simulink model "IKS02A1_VL53L1A1_Both_ROS_fromworkspace_2025b_forstudents"  (R2025b)
settings: Solver=FixedStepAuto  StartTime=0.0  StopTime=sensorLog.GT_time.time(end)  FixedStep=1/200  RelTol=1e-3
settings Model: Creator=abich  LastModifiedBy=ashra

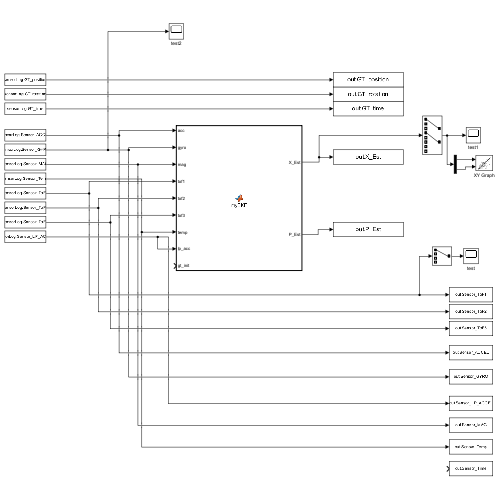
[thumbnail: Simulink's stored preview of the top-level diagram]
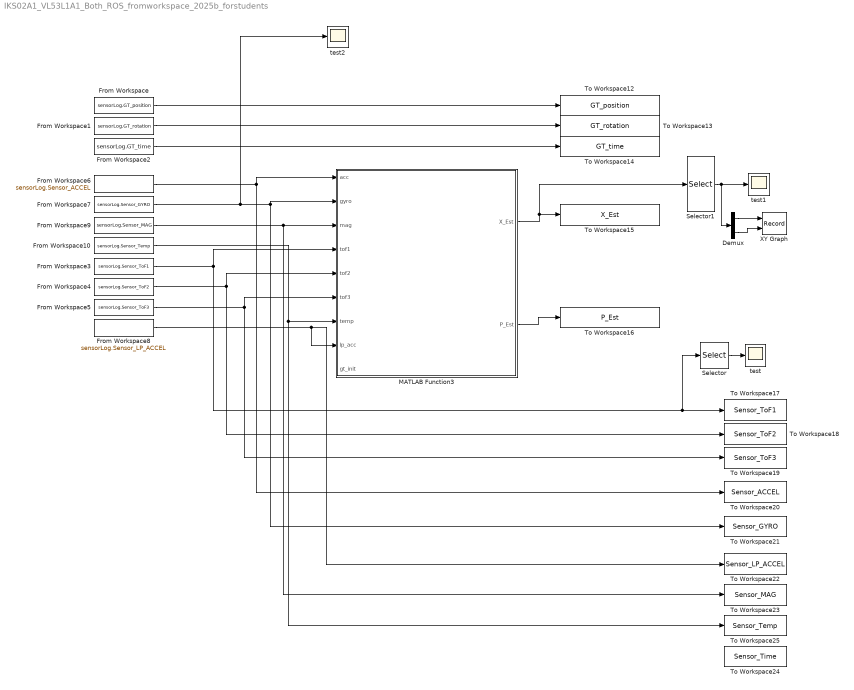
== system IKS02A1_VL53L1A1_Both_ROS_fromworkspace_2025b_forstudents ==
  Demux : Demux  Outputs=2
  From Workspace : FromWorkspace  VariableName=sensorLog.GT_position  SampleTime=1/200  OutputAfterFinalValue=Holding final value
  From Workspace1 : FromWorkspace  VariableName=sensorLog.GT_rotation  SampleTime=1/200  OutputAfterFinalValue=Holding final value
  From Workspace10 : FromWorkspace  VariableName=sensorLog.Sensor_Temp  SampleTime=1/200  OutputAfterFinalValue=Holding final value
  From Workspace2 : FromWorkspace  VariableName=sensorLog.GT_time  SampleTime=1/200  OutputAfterFinalValue=Holding final value
  From Workspace3 : FromWorkspace  VariableName=sensorLog.Sensor_ToF1  SampleTime=1/200  OutputAfterFinalValue=Holding final value
  From Workspace4 : FromWorkspace  VariableName=sensorLog.Sensor_ToF2  SampleTime=1/200  OutputAfterFinalValue=Holding final value
  From Workspace5 : FromWorkspace  VariableName=sensorLog.Sensor_ToF3  SampleTime=1/200  OutputAfterFinalValue=Holding final value
  From Workspace6 : FromWorkspace  VariableName=sensorLog.Sensor_ACCEL  SampleTime=1/200  OutputAfterFinalValue=Holding final value
  From Workspace7 : FromWorkspace  VariableName=sensorLog.Sensor_GYRO  SampleTime=1/200  OutputAfterFinalValue=Holding final value
  From Workspace8 : FromWorkspace  VariableName=sensorLog.Sensor_LP_ACCEL  SampleTime=1/200  OutputAfterFinalValue=Holding final value
  From Workspace9 : FromWorkspace  VariableName=sensorLog.Sensor_MAG  SampleTime=1/200  OutputAfterFinalValue=Holding final value
  MATLAB Function3 : MATLAB Function  TreatAsAtomicUnit=on
  Selector : Selector  InputPortWidth=4  IndexOptions=Index vector (dialog)  Indices=[1]  OutputSizes=1
  Selector1 : Selector  InputPortWidth=8  IndexOptions=Index vector (dialog)  Indices=[1 4]  OutputSizes=1
  To Workspace12 : ToWorkspace  VariableName=GT_position  SaveFormat=Structure With Time  SampleTime=1/200
  To Workspace13 : ToWorkspace  VariableName=GT_rotation  SaveFormat=Structure With Time  SampleTime=1/200
  To Workspace14 : ToWorkspace  VariableName=GT_time  SaveFormat=Structure With Time  SampleTime=1/200
  To Workspace15 : ToWorkspace  VariableName=X_Est  SaveFormat=Structure With Time  SampleTime=1/200
  To Workspace16 : ToWorkspace  VariableName=P_Est  SaveFormat=Structure With Time  SampleTime=1/200
  To Workspace17 : ToWorkspace  VariableName=Sensor_ToF1  SaveFormat=Structure With Time  SampleTime=1/200
  To Workspace18 : ToWorkspace  VariableName=Sensor_ToF2  SaveFormat=Structure With Time  SampleTime=1/200
  To Workspace19 : ToWorkspace  VariableName=Sensor_ToF3  SaveFormat=Structure With Time  SampleTime=1/200
  To Workspace20 : ToWorkspace  VariableName=Sensor_ACCEL  SaveFormat=Structure With Time  SampleTime=1/200
  To Workspace21 : ToWorkspace  VariableName=Sensor_GYRO  SaveFormat=Structure With Time  SampleTime=1/200
  To Workspace22 : ToWorkspace  VariableName=Sensor_LP_ACCEL  SaveFormat=Structure With Time  SampleTime=1/200
  To Workspace23 : ToWorkspace  VariableName=Sensor_MAG  SaveFormat=Structure With Time  SampleTime=1/200
  To Workspace24 : ToWorkspace  VariableName=Sensor_Time  SaveFormat=Structure With Time  SampleTime=1/200
  To Workspace25 : ToWorkspace  VariableName=Sensor_Temp  SaveFormat=Structure With Time  SampleTime=1/200
  XY Graph : Record  NumPorts=2.0  FileSettingsInternal="{\"entries\":[{\"content\":{\"excelSettings\":{\"content\":{},\"type\":\"Streamout.ExcelSettings\"},\"parquetSettings\":{\"content\":{},\"type\":\"Streamout.ParquetSettings\"}},\"type\":\"Streamout.FileSettingStorage\",\"uuid\":\"\"}],\"packageUris\":[\"http:\\/\\/schema.mathworks.com\\/mf0\\/streamout_blocks\\/R2020a\"],\"version\":\"1.0\"}"  FrameSettings=[0, 0]  Layout=[1 1]  SignalsInternal="{\"entries\":[{\"content\":{\"signals\":[{\"content\":{\"blockPath\":[],\"dimensions\":[1],\"domain\":\"\",\"lineColor\":\"#a2142f\",\"plots\":[ 1 ],\"port\":1,\"sid\":[\"\"],\"signalID\":1,\"signalName\":\"Demux:1\"},\"type\":\"RecordBlkView.Signal\",\"uuid\":\"\"},{\"content\":{\"blockPath\":[],\"dimensions\":[1],\"domain\":\"\",\"lineColor\":\"#139fff\",\"plots\":[ 1 ],\"port\":2,\"sid\":[\"\"],\"signalID\":2,\"signalName\":\"Demux:2\"},\"type\":\"RecordBlkView.Signal\",\"uuid\":\"\"}]},\"type\":\"RecordBlkView.InputSignals\",\"uuid\":\"\"}],\"packageUris\":[\"http:\\/\\/schema.mathworks.com\\/mf0\\/streamout_blocks\\/R2020a\"],\"version\":\"1.0\"}"  VisualizationBindings="{\"xyplotplugin\":{\"info\":[{\"series\":[{\"bindingParametersList\":[{\"parameter\":\"X-Axis\",\"signalID\":1,\"signalName\":\"Demux:1\"},{\"parameter\":\"Y-Axis\",\"signalID\":2,\"signalName\":\"Demux:2\"}],\"seriesID\":0}],\"subplotID\":1}]}}"  CompatibilityTag=XY
  test : Scope
      settings: ActiveDisplayYMinimum=-1  ActiveDisplayYMaximum=1
  test1 : Scope
      settings: ActiveDisplayYMinimum=-1.7865963660348574  ActiveDisplayYMaximum=1.7799074794929401
  test2 : Scope
      settings: ActiveDisplayYMinimum=-0.15108420974985681  ActiveDisplayYMaximum=0.16772460685752888  DataLoggingVariableName=ScopeData2
  wires:
  From Workspace4/1 -> To Workspace18/1, MATLAB Function3/5(tof2)
  From Workspace6/1 -> To Workspace20/1, MATLAB Function3/1(acc)
  From Workspace9/1 -> To Workspace23/1, MATLAB Function3/3(mag)
  From Workspace10/1 -> To Workspace25/1, MATLAB Function3/7(temp)
  From Workspace2/1 -> To Workspace14/1
  From Workspace5/1 -> To Workspace19/1, MATLAB Function3/6(tof3)
  From Workspace/1 -> To Workspace12/1
  MATLAB Function3/1(X_Est) -> Selector1/1, To Workspace15/1
  From Workspace8/1 -> To Workspace22/1, MATLAB Function3/8(lp_acc)
  From Workspace3/1 -> Selector/1, To Workspace17/1, MATLAB Function3/4(tof1)
  From Workspace1/1 -> To Workspace13/1
  From Workspace7/1 -> test2/1, To Workspace21/1, MATLAB Function3/2(gyro)
  MATLAB Function3/2(P_Est) -> To Workspace16/1
  Selector/1 -> test/1
  Selector1/1 -> Demux/1, test1/1
  Demux/1 -> XY Graph/1
  Demux/2 -> XY Graph/2

== matlab function IKS02A1_VL53L1A1_Both_ROS_fromworkspace_2025b_forstudents/MATLAB Function3 ==
  data: acc input; X_Est output; gyro input; mag input; tof1 input; tof2 input; tof3 input; P_Est output; temp input; lp_acc input; gt_init input
function [X_Est, P_Est] = myEKF(acc, gyro, mag, tof1, tof2, tof3, temp, lp_acc, gt_init)
% CALLING CONVENTION:
%   First call:  myEKF(acc,gyro,mag,tof1,tof2,tof3,temp,lp_acc,[x0,y0,theta0])
%   All others:  myEKF(acc,gyro,mag,tof1,tof2,tof3,temp,lp_acc)
%
% STATE VECTOR (world frame):
%   x_state = [x, vx, ax,  y, vy, ay,  theta, omega]
%              1   2   3   4   5   6      7      8
%
% =========================================================================


persistent x_state P arena ...
    GYRO_Z_IDX GYRO_Z_SIGN gyro_bias_z R_gyro OMEGA_STILL_THRESH ...
    ACCEL_X_IDX ACCEL_X_SIGN ACCEL_BIAS_X ...
    ACCEL_Y_IDX ACCEL_Y_SIGN ACCEL_BIAS_Y ...
    sensors Q R_accel R_tof ...
    MAG_FUNCTIONAL mag_hard_iron mag_soft_iron mag_yaw_offset R_mag ...
    still_counter reacq_fired is_init sample_count ...
    prev_tof USE_GT_INIT tof_age ...
    heading_refine_tof heading_refine_count heading_refined

if nargin < 9; gt_init = []; end


%  ONE-TIME SETUP — runs only on the very first call each simulation
% =========================================================================
if isempty(is_init)

    % --- Arena bounds [m] ---
    arena.x_min = -1.22;  arena.x_max = 1.22;
    arena.y_min = -1.22;  arena.y_max = 1.22;

    % -----------------------------------------------------------------
    %  GYRO

    GYRO_Z_IDX        = 1;       
    GYRO_Z_SIGN       = +1;        
    gyro_bias_z       = 0.001883; % [rad/s] static bias
    R_gyro            = (0.005)^2;% measurement noise variance
    OMEGA_STILL_THRESH = 0.08;    % [rad/s]

    % -----------------------------------------------------------------

    %  ACCELEROMETER

    ACCEL_X_IDX  = 3;        % forward axis column
    ACCEL_X_SIGN = +1;
    ACCEL_BIAS_X = -0.3962;  
    ACCEL_Y_IDX  = 2;        % lateral axis column
    ACCEL_Y_SIGN = +1;
    ACCEL_BIAS_Y =  0.0278;  
    R_accel      = (1.02)^2;

    sensors = repmat(struct('angle_offset', 0, 'offset_x', 0, 'offset_y', 0), 3, 1);
    sensors(1).angle_offset =  pi/2;   % ToF1 -> Left
    sensors(1).offset_x = 0;  sensors(1).offset_y =  0;
    sensors(2).angle_offset =  pi;     % ToF2 -> Backward
    sensors(2).offset_x = 0;  sensors(2).offset_y =  0;
    sensors(3).angle_offset = -pi/2;   % ToF3 -> Right
    sensors(3).offset_x = 0;  sensors(3).offset_y = 0;
    R_tof =  0.02;

    % -----------------------------------------------------------------
    %  MAGNETOMETER: We found using the magnetometer creating lots of
    %  issues due to its resolution so we have had to dissable it but our
    %  implementation is still here.
    %
    %  The update is gated: it only fires when omega < MAG_UPDATE_OMEGA_MAX
    %  so it does not try to correct heading mid-spin.
    %
    % -----------------------------------------------------------------
    MAG_FUNCTIONAL   = false;    % disabled: 78 deg std makes it harmful
    mag_hard_iron    = [1.470000e-05, -4.020000e-05]; 
    mag_soft_iron    = [2.340000e-05, 2.370000e-05];   
    mag_yaw_offset   = -0.1017;             
    R_mag            = 1.8646;             

    % -----------------------------------------------------------------
    %  PROCESS NOISE COVARIANCE Q
    %  Larger values = trust the motion model less (accel noise dominates).
    % -----------------------------------------------------------------
    Q = zeros(8,8);
    Q(1,1) = 0.005;    % x position
    Q(2,2) = 0.05;     % x velocity (higher = adapts faster to motion)
    Q(3,3) = 3;        % x acceleration (large: accel model is rough)
    Q(4,4) = 0.005;    % y position
    Q(5,5) = 0.05;     % y velocity
    Q(6,6) = 3;        % y acceleration
    Q(7,7) = 0.01;     % heading
    Q(8,8) = 0.01;     % angular rate

    % -----------------------------------------------------------------
    %  INITIALISATION MODE
    %  USE_GT_INIT = true  → use ground-truth position (for testing)
    %  USE_GT_INIT = false → assume start at middle of left wall (for
    %                        assessment)
    % -----------------------------------------------------------------
    USE_GT_INIT = true;   % FLIP TO false for the assessment

    % -----------------------------------------------------------------
    %  INITIAL STATE & COVARIANCE
    % -----------------------------------------------------------------
    x_state       = zeros(8,1);
    P             = diag([0.5, 1.0, 4.0, 0.5, 1.0, 4.0, 0.5, 1.0]);
    still_counter = 0;
    reacq_fired   = false;
    sample_count  = 0;
    prev_tof      = nan(1,3);   
    tof_age       = 999;        
    heading_refine_tof = zeros(5,3);  
    heading_refine_count = 0;
    heading_refined = false;
    is_init       = true;
end

sample_count = sample_count + 1;
dt = 1 / 200;   % All signals logged at 200 Hz in Simulink


if sample_count == 1
    tof_z = read_tof(tof1, tof2, tof3);

    if USE_GT_INIT && ~isempty(gt_init) && numel(gt_init) >= 3
        % --- Mode A: GT-seeded position ---
        x_state(1) = gt_init(1);   % x [m]
        x_state(4) = gt_init(2);   % y [m]
        P(1,1) = 0.005;
        P(4,4) = 0.005;

        x_state(7) = heading_scan_full(gt_init(1), gt_init(2), tof_z, ...
                                        gt_init(3), sensors, arena);
        P(7,7) = (5*pi/180)^2;

        fprintf('=== EKF INIT (GT mode) ===\n');
        fprintf('  pos=(%.3f, %.3f)  theta_quat=%.1f deg  theta_scan=%.1f deg\n', ...
            gt_init(1), gt_init(2), rad2deg(gt_init(3)), rad2deg(x_state(7)));

    else
        % --- Mode B: Blind init — middle of left wall ---
        wall_offset = 0.05;   % [m] small offset from wall surface
        x_state(1) = arena.x_min + wall_offset;   % x near left wall
        x_state(4) = 0;                            % y = arena centre
        P(1,1) = 0.02;    % fairly confident in x (touching wall)
        P(4,4) = 0.5;     % less sure about y along the wall

        % Heading scan: no GT hint, search full 360
        x_state(7) = heading_scan_full(x_state(1), x_state(4), tof_z, ...
                                        0, sensors, arena);
        P(7,7) = (10*pi/180)^2;   % wider uncertainty without GT hint

        fprintf('=== EKF INIT (BLIND mode — left wall) ===\n');
        fprintf('  pos=(%.3f, %.3f)  theta_scan=%.1f deg\n', ...
            x_state(1), x_state(4), rad2deg(x_state(7)));
    end

    fprintf('  tof=[%.3f %.3f %.3f]\n', tof_z(1), tof_z(2), tof_z(3));
    
    fprintf('================\n');
end

% =========================================================================
%  PREDICTION STEP  (constant-acceleration kinematic model)
% =========================================================================
% Velocity damping factor: models friction / drag so velocity decays
% when acceleration drops.  alpha=0.98 means ~2% decay per 5ms step.

alpha_v = 0.99;   % velocity damping per step
F = [1, dt, 0.5*dt^2, 0,  0,        0, 0,   0;
     0,  alpha_v,  dt, 0,  0,        0, 0,   0;
     0,  0,        1, 0,  0,        0, 0,   0;
     0,  0,        0, 1, dt, 0.5*dt^2, 0,   0;
     0,  0,        0, 0, alpha_v,  dt, 0,   0;
     0,  0,        0, 0,  0,        1, 0,   0;
     0,  0,        0, 0,  0,        0, 1,  dt;
     0,  0,        0, 0,  0,        0, 0,   1];

x_pred = F * x_state;
P_pred = F * P * F' + Q;

% =========================================================================
%  GYRO UPDATE

omega_for_gate = 0;   % used later for motion gating
if ~any(isnan(gyro))
    omega_raw   = GYRO_Z_SIGN * double(gyro(GYRO_Z_IDX));
    omega_meas  = omega_raw - gyro_bias_z;
    H_gyro      = [0,0,0, 0,0,0, 0,1];
    [x_pred, P_pred] = ekf_update(x_pred, P_pred, omega_meas, x_pred(8), ...
                                   H_gyro, R_gyro);

    % Use max of all columns for motion gating — guards against axes where
    % one column reads near-zero during actual yaw rotations.
    omega_for_gate = max(abs(double(gyro)));

    % Per-second diagnostic log
    if mod(sample_count, 200) == 0
        fprintf('[t=%5.1fs] gyro_raw=[%+.4f %+.4f %+.4f]  omega=%.4f  theta=%+.1f deg\n', ...
            sample_count/200, gyro(1), gyro(2), gyro(3), omega_meas, rad2deg(x_pred(7)));
    end
end

% =========================================================================
%  MAGNETOMETER UPDATE

MAG_UPDATE_OMEGA_MAX = 0.15;   % [rad/s] — tune if mag causes jitter

if MAG_FUNCTIONAL && ~any(isnan(mag)) && omega_for_gate < MAG_UPDATE_OMEGA_MAX
    Mx = double(mag(1));
    My = double(mag(2));

    % Hard-iron then soft-iron correction
    Mx_cal = (Mx - mag_hard_iron(1)) / mag_soft_iron(1);
    My_cal = (My - mag_hard_iron(2)) / mag_soft_iron(2);

    % Derive heading from horizontal mag field
    z_mag = wrap_angle(atan2(My_cal, Mx_cal) + mag_yaw_offset);

    % Innovation — must be angle-wrapped to avoid 2pi jumps
    innov_mag = wrap_angle(z_mag - x_pred(7));

    % EKF update manually (standard linear update, but wrapping innovation)
    H_mag = [0,0,0, 0,0,0, 1,0];
    S_mag = H_mag * P_pred * H_mag' + R_mag;
    K_mag = P_pred * H_mag' / S_mag;
    x_pred = x_pred + K_mag * innov_mag;
    x_pred(7) = wrap_angle(x_pred(7));
    P_pred = (eye(8) - K_mag * H_mag) * P_pred;
end

% =========================================================================
%  ACCELEROMETER UPDATE

if ~any(isnan(acc))
    ax_body  = ACCEL_X_SIGN * (double(acc(ACCEL_X_IDX)) - ACCEL_BIAS_X);
    ay_body  = ACCEL_Y_SIGN * (double(acc(ACCEL_Y_IDX)) - ACCEL_BIAS_Y);
    c = cos(x_pred(7));  s = sin(x_pred(7));
    ax_world =  c*ax_body - s*ay_body;
    ay_world =  s*ax_body + c*ay_body;
    [x_pred, P_pred] = ekf_update(x_pred, P_pred, ax_world, x_pred(3), ...
                                   [0,0,1, 0,0,0, 0,0], R_accel);
    [x_pred, P_pred] = ekf_update(x_pred, P_pred, ay_world, x_pred(6), ...
                                   [0,0,0, 0,0,1, 0,0], R_accel);
end

% =========================================================================
%  ToF UPDATES
%
%  Corrects position (x, y) ONLY.  H_tof(7) and H_tof(8) are zeroed so
%  ToF never directly corrects heading.  Heading is gyro's job; ToF's job
%  is position.  Mixing them causes heading/position feedback loops.
%
%  GATING:
%    - Valid reading: status=0, range in [0.05, 2.5] m
%    - Not spinning fast (|omega| <= 1.0 rad/s)
%    - Innovation within 3-sigma gate
% =========================================================================
tof_inputs = {tof1, tof2, tof3};
tof_changed = false;   % track if any ToF reading changed (robot moving)
tof_age = tof_age + 1; % increment age; reset below if any ToF changes
for s_idx = 1:3
    td = tof_inputs{s_idx};
    if any(isnan(td));               continue; end
    if td(4) ~= 0;                   continue; end
    z_tof = double(td(1));
    if isnan(z_tof) || isinf(z_tof); continue; end
    if z_tof < 0.05 || z_tof > 2.5; continue; end
    if abs(x_pred(8)) > 0.3;         continue; end   % skip during turns (wall holes)
    % Skip duplicate readings (same value = zero-order hold, not new data)
    if z_tof == prev_tof(s_idx);     continue; end
    tof_changed = true;
    tof_age = 0;              % reset: ToF just changed
    prev_tof(s_idx) = z_tof;
    % Signal-strength filter: low signal = through wall hole or bad reading
    sig = double(td(3));
    if sig < 300;                     continue; end

    h_val = h_tof_sensor(x_pred, sensors(s_idx), arena);
    if isinf(h_val) || isnan(h_val); continue; end

    H_tof_raw = compute_H_tof_numerical(x_pred, sensors(s_idx), arena, 1e-6);
    H_tof     = [H_tof_raw(1:6), 0, 0];

    S_tof = H_tof * P_pred * H_tof' + R_tof;
    innov = z_tof - h_val;

    gate = min(3*sqrt(S_tof), 0.8);   % 3-sigma, cap at 0.8 m
    if abs(innov) > gate;              continue; end

    K_tof  = P_pred * H_tof' / S_tof;
    x_pred = x_pred + K_tof * innov;
    x_pred(7) = wrap_angle(x_pred(7));
    P_pred = (eye(8) - K_tof*H_tof) * P_pred;
end

% =========================================================================
%  HEADING REFINEMENT (first 0.5s only)
%  Collect first 5 unique ToF readings, then re-do heading scan with the
%  median values — reduces noise from a single ToF snapshot at init.
% =========================================================================
if ~heading_refined && tof_changed && omega_for_gate < OMEGA_STILL_THRESH
    heading_refine_count = heading_refine_count + 1;
    tof_now = read_tof(tof1, tof2, tof3);
    if heading_refine_count <= 5
        heading_refine_tof(heading_refine_count,:) = tof_now;
    end
    if heading_refine_count == 5
        % Use median of 5 readings for a more robust heading scan
        med_tof = median(heading_refine_tof, 1);
        % Only refine if all 3 sensors have valid median
        if ~any(isnan(med_tof))
            new_theta = heading_scan_full(x_pred(1), x_pred(4), med_tof, ...
                                           x_pred(7), sensors, arena);
            % Only accept if within 15 deg of current (sanity check)
            if abs(wrap_angle(new_theta - x_pred(7))) < deg2rad(15)
                x_pred(7) = new_theta;
                P_pred(7,7) = (3*pi/180)^2;  % tighter heading uncertainty
            end
        end
        heading_refined = true;
    end
end

% =========================================================================

if omega_for_gate > OMEGA_STILL_THRESH
    still_counter = 0;
    reacq_fired   = false;
else
    still_counter = still_counter + 1;
end

% =========================================================================
%  ZERO-VELOCITY UPDATE (ZUPT)
%
%  When all gyro axes are quiet AND acceleration is near its stationary
%  value, the robot is not moving.  Inject vx=0, vy=0 measurements to
%  kill residual velocity from the motion model.

ZUPT_R = 0.001;  % velocity measurement noise [m/s]^2
ZAUT_R = 0.1;    % acceleration measurement noise [m/s^2]^2
if omega_for_gate < OMEGA_STILL_THRESH && tof_age > 40
    % Only ZUPT when gyro quiet AND ToF hasn't changed for >40 samples
    % (0.2s = 2 ToF cycles).  During constant-velocity motion, ToF readings
    % keep changing every ~20 samples — tof_age stays low, blocking ZUPT.
    if ~any(isnan(acc))
        grav_dev = abs(double(acc(1)) - 10.0);
        fwd_dev  = abs(double(acc(ACCEL_X_IDX)) - ACCEL_BIAS_X);
        lat_dev  = abs(double(acc(ACCEL_Y_IDX)) - ACCEL_BIAS_Y);
        if grav_dev < 0.5 && fwd_dev < 0.4 && lat_dev < 0.4  % all axes quiet
            % Zero-velocity update
            [x_pred, P_pred] = ekf_update(x_pred, P_pred, 0, x_pred(2), ...
                                           [0,1,0, 0,0,0, 0,0], ZUPT_R);
            [x_pred, P_pred] = ekf_update(x_pred, P_pred, 0, x_pred(5), ...
                                           [0,0,0, 0,1,0, 0,0], ZUPT_R);
            % Zero-acceleration update
            [x_pred, P_pred] = ekf_update(x_pred, P_pred, 0, x_pred(3), ...
                                           [0,0,1, 0,0,0, 0,0], ZAUT_R);
            [x_pred, P_pred] = ekf_update(x_pred, P_pred, 0, x_pred(6), ...
                                           [0,0,0, 0,0,1, 0,0], ZAUT_R);
        end
    end
end

% =========================================================================
%  STATE / COVARIANCE CLIPPING
% =========================================================================
x_pred(1) = max(arena.x_min+0.05, min(arena.x_max-0.05, x_pred(1)));
x_pred(4) = max(arena.y_min+0.05, min(arena.y_max-0.05, x_pred(4)));
x_pred(2) = max(-1.5, min(1.5, x_pred(2)));
x_pred(5) = max(-1.5, min(1.5, x_pred(5)));
x_pred(8) = max(-5.0, min(5.0, x_pred(8)));
x_pred(7) = wrap_angle(x_pred(7));
P_pred    = 0.5*(P_pred + P_pred');   % enforce symmetry

x_state = x_pred;
P       = P_pred;
X_Est   = x_state;
P_Est   = P;

end  % ← end myEKF


% =========================================================================
%  HEADING SCAN HELPERS
% =========================================================================

function best_theta = heading_scan_full(px, py, tof_z, theta_fallback, sensors, arena)
    % Two-pass heading scan: coarse (1 deg) then fine (0.05 deg) around best.
    % Pass 1: coarse scan
    N_coarse = 360;
    theta_coarse = linspace(-pi, pi, N_coarse+1);
    theta_coarse = theta_coarse(1:N_coarse);
    best_theta  = theta_fallback;
    best_n      = -1;
    best_sse    = Inf;
    for tc = 1:N_coarse
        th     = theta_coarse(tc);
        x_cand = zeros(8,1);
        x_cand(1) = px;  x_cand(4) = py;  x_cand(7) = th;
        n = 0;  sse = 0;
        for si = 1:3
            if isnan(tof_z(si)); continue; end
            h = h_tof_sensor(x_cand, sensors(si), arena);
            if isinf(h) || isnan(h); continue; end
            innov = tof_z(si) - h;
            if abs(innov) < 0.5
                n = n+1;  sse = sse+innov^2;
            end
        end
        if n > best_n || (n == best_n && sse < best_sse)
            best_n = n;  best_sse = sse;  best_theta = th;
        end
    end
    % Pass 2: fine scan ±3 deg around coarse best (0.05 deg steps)
    fine_range = deg2rad(3);
    N_fine = 120;
    theta_fine = linspace(best_theta - fine_range, best_theta + fine_range, N_fine+1);
    for tc = 1:N_fine+1
        th     = theta_fine(tc);
        x_cand = zeros(8,1);
        x_cand(1) = px;  x_cand(4) = py;  x_cand(7) = th;
        n = 0;  sse = 0;
        for si = 1:3
            if isnan(tof_z(si)); continue; end
            h = h_tof_sensor(x_cand, sensors(si), arena);
            if isinf(h) || isnan(h); continue; end
            innov = tof_z(si) - h;
            if abs(innov) < 0.5
                n = n+1;  sse = sse+innov^2;
            end
        end
        if n > best_n || (n == best_n && sse < best_sse)
            best_n = n;  best_sse = sse;  best_theta = th;
        end
    end
    best_theta = wrap_angle(best_theta);
end

function theta_out = heading_scan_constrained(px, py, tof_z, theta_current, ...
                                               sensors, arena, max_dev, min_ratio)
    % Constrained scan — only considers headings within max_dev of current.
    % Accepts new heading only if SSE improves by factor min_ratio.
    N_cands = 360;
    theta_cands = linspace(-pi, pi, N_cands+1);
    theta_cands = theta_cands(1:N_cands);
    best_theta  = theta_current;
    best_score  = Inf;

    x_cur        = zeros(8,1);
    x_cur(1) = px;  x_cur(4) = py;  x_cur(7) = theta_current;
    baseline = tof_sse(x_cur, tof_z, sensors, arena);

    for tc = 1:N_cands
        th = theta_cands(tc);
        if abs(wrap_angle(th - theta_current)) > max_dev; continue; end
        x_cand    = zeros(8,1);
        x_cand(1) = px;  x_cand(4) = py;  x_cand(7) = th;
        s = tof_sse(x_cand, tof_z, sensors, arena);
        if s < best_score;  best_score = s;  best_theta = th;  end
    end

    if isfinite(best_score) && best_score < baseline / min_ratio
        theta_out = wrap_angle(best_theta);
    else
        theta_out = theta_current;
    end
end

function s = tof_sse(x8, tof_z, sensors, arena)
    n = 0;  sse = 0;
    for si = 1:3
        if isnan(tof_z(si)); continue; end
        h = h_tof_sensor(x8, sensors(si), arena);
        if isinf(h) || isnan(h); continue; end
        innov = tof_z(si) - h;
        if abs(innov) < 0.5;  n = n+1;  sse = sse+innov^2;  end
    end
    if n == 0;  s = Inf;  else;  s = sse/n;  end
end

function tof_z = read_tof(tof1, tof2, tof3)
    % Return [d1, d2, d3]; NaN if reading invalid.
    tof_z = nan(1,3);
    raw   = {tof1, tof2, tof3};
    for si = 1:3
        td = raw{si};
        if ~any(isnan(td)) && td(4)==0 && td(1)>=0.05 && td(1)<=2.5
            tof_z(si) = double(td(1));
        end
    end
end


% =========================================================================
%  EKF CORE HELPERS
% =========================================================================

function [x_out, P_out] = ekf_update(x_in, P_in, z, h_val, H, R)
    % Standard linear EKF update.
    innov = z - h_val;
    S     = H * P_in * H' + R;
    K     = P_in * H' / S;
    x_out = x_in + K * innov;
    P_out = (eye(length(x_in)) - K*H) * P_in;
end

function d = h_tof_sensor(x_state, sensor, arena)
    % Predicted distance from (sensor position) in (sensor direction) to wall.
    x = x_state(1);  y = x_state(4);  theta = x_state(7);
    c = cos(theta);  s = sin(theta);
    % Sensor position in world frame (accounting for body-frame offset)
    xs = x + sensor.offset_x*c - sensor.offset_y*s;
    ys = y + sensor.offset_x*s + sensor.offset_y*c;
    ra  = theta + sensor.angle_offset;
    rdx = cos(ra);  rdy = sin(ra);
    eps = 1e-6;  dists = [];
    if abs(rdx) > eps
        t = (arena.x_max - xs)/rdx;
        if t>eps && inrange(ys+t*rdy, arena.y_min, arena.y_max, eps); dists(end+1)=t; end
        t = (arena.x_min - xs)/rdx;
        if t>eps && inrange(ys+t*rdy, arena.y_min, arena.y_max, eps); dists(end+1)=t; end
    end
    if abs(rdy) > eps
        t = (arena.y_max - ys)/rdy;
        if t>eps && inrange(xs+t*rdx, arena.x_min, arena.x_max, eps); dists(end+1)=t; end
        t = (arena.y_min - ys)/rdy;
        if t>eps && inrange(xs+t*rdx, arena.x_min, arena.x_max, eps); dists(end+1)=t; end
    end
    if isempty(dists);  d = Inf;  else;  d = min(dists);  end
end

function ok = inrange(v, lo, hi, eps)
    ok = v >= lo-eps && v <= hi+eps;
end

function H = compute_H_tof_numerical(x_state, sensor, arena, ev)
    % Numerical Jacobian for ToF measurement.
    H  = zeros(1,8);
    h0 = h_tof_sensor(x_state, sensor, arena);
    if isinf(h0);  return;  end
    for idx = [1, 4, 7]    % only x, y, theta matter
        xp = x_state;  xp(idx) = xp(idx) + ev;
        xm = x_state;  xm(idx) = xm(idx) - ev;
        hp = h_tof_sensor(xp, sensor, arena);
        hm = h_tof_sensor(xm, sensor, arena);
        if ~isinf(hp) && ~isinf(hm)
            H(idx) = (hp - hm) / (2*ev);
        end
    end
end

function a = wrap_angle(a)
    a = mod(a + pi, 2*pi) - pi;
end
